simulink model "Wiper_StateFlow"  (R2016a)
settings: Solver=FixedStepAuto  StartTime=0.0  StopTime=9  FixedStep=Tsample  RelTol=1e-3
undefined symbols (not defined in the file or in its folder): LeftPosition, ON_High, ON_Low, ON_Normal, RainSens_High, RainSens_Low, RightPosition, Tsample, WiCmd_High, WiCmd_Low, WiCmd_Max, WiCmd_Normal
libraries: sh_lib x1
settings Model: Creator=Cosmin  LastModifiedBy=Cosmin

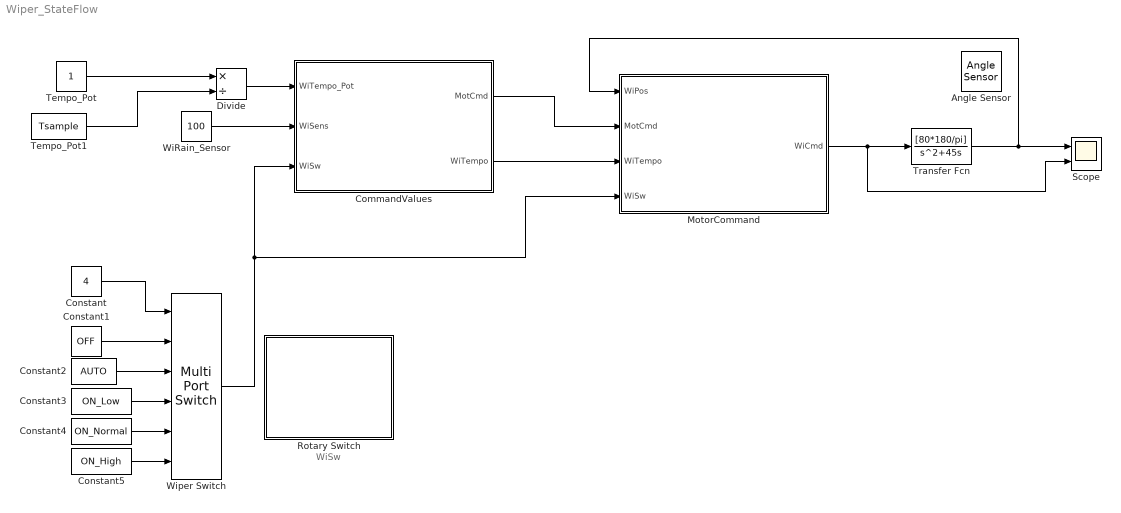
== system Wiper_StateFlow ==
  note: WiSw
  Angle Sensor : sh_lib/Pumps and Motors/Angle Sensor  phase_angle=0 rad
  CommandValues : Stateflow chart  TreatAsAtomicUnit=on
  Constant : Constant  Value=4
  Constant1 : Constant  Value=OFF
  Constant2 : Constant  Value=AUTO
  Constant3 : Constant  Value=ON_Low
  Constant4 : Constant  Value=ON_Normal
  Constant5 : Constant  Value=ON_High
  Divide : Product  Inputs=*/
  MotorCommand : Stateflow chart  TreatAsAtomicUnit=on
  Rotary Switch : Subsystem  DialogController=hmiCreateDDGDialog  IsWebBlock=on  mask(MWDashboardBlock){webBlockId=043e65d8-e32a-48b2-a02b-e0f434f003c5, webBlockType=discreteknob, ShowInLibBrowser=on, ShowInitialText=on, HMISrcModelName=Wiper_StateFlow}
      mask prompts: webBlockId "WebBlock Id"; webBlockType "WebBlock Type"; HMISrcModelName "Source Model"
      mask Help: helpview([docroot '/mapfiles/simulink.map'], 'hmi_rotary_switch')
      mask Display:
      | model = bdroot(gcb);
      | if strcmp(get_param(model,'BlockDiagramType'), 'library')
      |     image([(matlabroot) '/toolbox/simulink/hmi/icons/DiscreteKnob.png']);
      | end
  Scope : Scope  NumInputPorts=2
  Tempo_Pot : Constant
  Tempo_Pot1 : Constant  Value=Tsample
  Transfer Fcn : TransferFcn  Numerator=[80*180/pi]  Denominator=[1 45 0]
  WiRain_Sensor : Constant  Value=100
  Wiper Switch : MultiPortSwitch  DataPortOrder=Zero-based contiguous  Inputs=5
  wires:
  Transfer Fcn/1 -> Scope/1, MotorCommand/1(WiPos)
  MotorCommand/1(WiCmd) -> Scope/2, Transfer Fcn/1
  CommandValues/1(MotCmd) -> MotorCommand/2(MotCmd)
  CommandValues/2(WiTempo) -> MotorCommand/3(WiTempo)
  Wiper Switch/1 -> MotorCommand/4(WiSw), CommandValues/3(WiSw)
  Constant/1 -> Wiper Switch/1
  Constant1/1 -> Wiper Switch/2
  Constant2/1 -> Wiper Switch/3
  Constant3/1 -> Wiper Switch/4
  Constant4/1 -> Wiper Switch/5
  Constant5/1 -> Wiper Switch/6
  WiRain_Sensor/1 -> CommandValues/2(WiSens)
  Divide/1 -> CommandValues/1(WiTempo_Pot)
  Tempo_Pot/1 -> Divide/1
  Tempo_Pot1/1 -> Divide/2

== system Wiper_StateFlow/Rotary Switch ==

== stateflow chart Wiper_StateFlow/CommandValues ==
  (default) -> (junction 2)
  (junction 2) -> (junction 3) [order 1] : [WiSw==OFF]{MotCmd=OFF;WiTempo=0;}
  (junction 14) -> (junction 16) [order 1] : [WiSw==ON_Low]...
      | {MotCmd=WiCmd_Low;WiTempo=WiTempo_Pot;}
  (junction 2) -> (junction 14) [order 3]
  (junction 2) -> (junction 6) [order 2] : [WiSw==AUTO]
  (junction 14) -> (junction 17) [order 2] : [WiSw==ON_Normal]...
      | {MotCmd=WiCmd_Normal;WiTempo=0;}
  (junction 14) -> (junction 18) [order 3] : [WiSw==ON_High]...
      | {MotCmd=WiCmd_High;WiTempo=0;}
  (junction 6) -> (junction 8) [order 1] : [WiSens<RainSens_Low]{MotCmd=OFF;WiTempo=0;}
  (junction 6) -> (junction 12) [order 3] : [WiSens>RainSens_High]...
      | {MotCmd = WiCmd_Normal + (WiSens - RainSens_High) * (WiCmd_Max - WiCmd_Normal)/(100 - RainSens_High);...
      | WiTempo=0;}
  (junction 6) -> (junction 10) [order 2] : [(WiSens>=RainSens_Low)&&(WiSens<=RainSens_High)]...
      | {MotCmd = WiCmd_Low+(WiSens-RainSens_Low)*(WiCmd_Normal-WiCmd_Low)/(RainSens_High-RainSens_Low);...
      | WiTempo=WiTempo_Pot-(WiSens-RainSens_Low)*WiTempo_Pot/(RainSens_High-RainSens_Low);}
  data: WiCmd_Low parameter; WiCmd_High parameter; WiTempo_Pot input; WiSens input; RainSens_Low parameter; WiSw input; ON_Low parameter; RainSens_High parameter; WiCmd_Normal parameter; ON_Normal parameter; MotCmd output; WiTempo output; OFF parameter; AUTO parameter; WiCmd_Max parameter; ON_High parameter

== stateflow chart Wiper_StateFlow/MotorCommand ==
  state Left
    en: WiCmd=MotCmd;
  state Right
    en: WiCmd=-MotCmd;
  state Tempo
    en: WiCmd=0;
    timp=0;
    du: timp=timp+1;
  (default) -> (junction 2)
  (junction 2) -> (junction 3) [order 1] : [WiSw==OFF]{WiCmd=0;}
  (junction 2) -> Left [order 2]
  Left -> Right : [WiPos>LeftPosition]
  (junction 13) -> Left [order 1] : [WiTempo==0]
  Tempo -> Left : [timp>=WiTempo]
  Right -> (junction 13) : [WiPos<=RightPosition]
  (junction 13) -> Tempo [order 2]
  data: WiPos input; LeftPosition parameter; RightPosition parameter; MotCmd input; WiTempo input; WiSw input; WiCmd output; timp local; OFF parameter
